simulink model "Tires"  (R2023a)
settings: Solver=VariableStepAuto  StartTime=0.0  StopTime=10.0  RelTol=1e-3
undefined symbols (not defined in the file): C, C_alpha_f, C_r, E, e_p0, F_zf, l_f, l_r, n_st
settings Model: Creator=Tan_Tram  LastModifiedBy=Tan_Tram

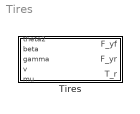
== system Tires ==
  Tires : Subsystem

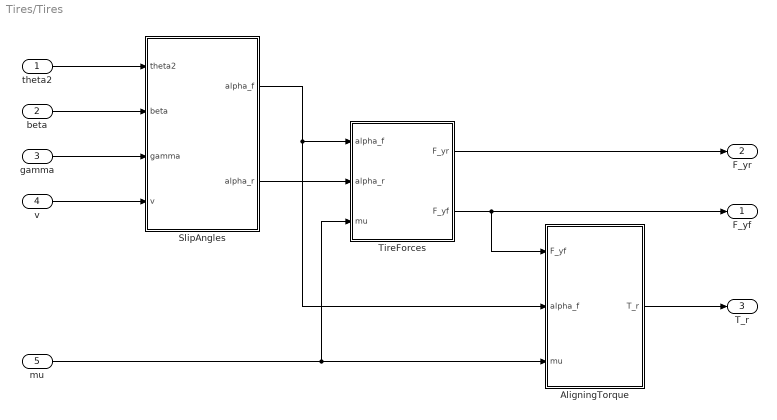
== system Tires/Tires ==
  theta2 : Inport
  beta : Inport  Port=2
  gamma : Inport  Port=3
  v : Inport  Port=4
  mu : Inport  Port=5
  AligningTorque : Subsystem
  SlipAngles : Subsystem
  TireForces : Subsystem
  F_yf : Outport
  F_yr : Outport  Port=2
  T_r : Outport  Port=3
  wires:
  v/1 -> SlipAngles/4(v)
  gamma/1 -> SlipAngles/3(gamma)
  TireForces/2(F_yf) -> F_yf/1, AligningTorque/1(F_yf)
  beta/1 -> SlipAngles/2(beta)
  theta2/1 -> SlipAngles/1(theta2)
  SlipAngles/2(alpha_r) -> TireForces/2(alpha_r)
  SlipAngles/1(alpha_f) -> TireForces/1(alpha_f), AligningTorque/2(alpha_f)
  mu/1 -> AligningTorque/3(mu), TireForces/3(mu)
  TireForces/1(F_yr) -> F_yr/1
  AligningTorque/1(T_r) -> T_r/1

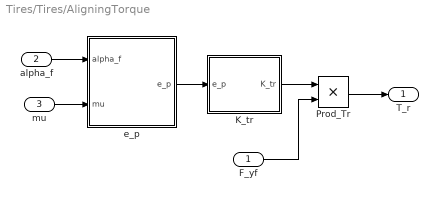
== system Tires/Tires/AligningTorque ==
  F_yf : Inport
  alpha_f : Inport  Port=2
  mu : Inport  Port=3
  K_tr : Subsystem
  Prod_Tr : Product  Inputs=**
  e_p : Subsystem
  T_r : Outport
  wires:
  F_yf/1 -> Prod_Tr/2
  Prod_Tr/1 -> T_r/1
  alpha_f/1 -> e_p/1(alpha_f)
  mu/1 -> e_p/2(mu)
  e_p/1(e_p) -> K_tr/1(e_p)
  K_tr/1(K_tr) -> Prod_Tr/1

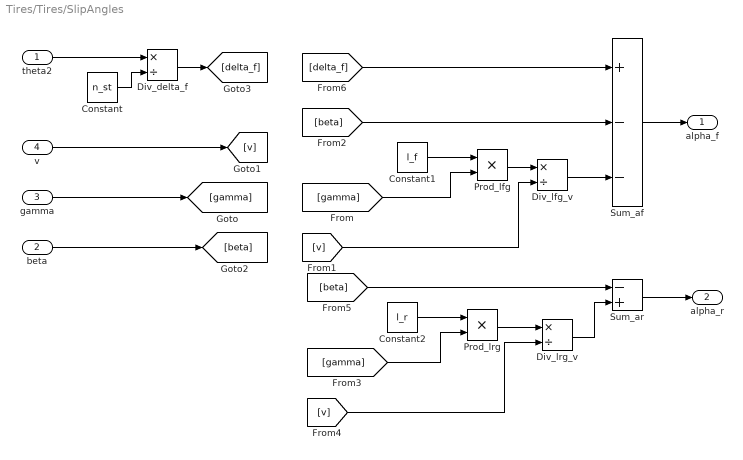
== system Tires/Tires/SlipAngles ==
  theta2 : Inport
  beta : Inport  Port=2
  gamma : Inport  Port=3
  v : Inport  Port=4
  Constant : Constant  Value=n_st
  Constant1 : Constant  Value=l_f
  Constant2 : Constant  Value=l_r
  Div_delta_f : Product  Inputs=*/
  Div_lfg_v : Product  Inputs=*/
  Div_lrg_v : Product  Inputs=*/
  Prod_lfg : Product  Inputs=**
  Prod_lrg : Product  Inputs=**
  Sum_af : Sum  Inputs=+--
  Sum_ar : Sum  Inputs=-+
  alpha_f : Outport
  alpha_r : Outport  Port=2
  wires:
  beta/1 -> [beta]
  Div_lrg_v/1 -> Sum_ar/2
  Constant2/1 -> Prod_lrg/1
  Div_lfg_v/1 -> Sum_af/3
  Constant1/1 -> Prod_lfg/1
  gamma/1 -> [gamma]
  [gamma] -> Prod_lfg/2
  v/1 -> [v]
  [gamma] -> Prod_lrg/2
  Sum_ar/1 -> alpha_r/1
  [v] -> Div_lrg_v/2
  Prod_lfg/1 -> Div_lfg_v/1
  [v] -> Div_lfg_v/2
  Prod_lrg/1 -> Div_lrg_v/1
  Sum_af/1 -> alpha_f/1
  [beta] -> Sum_af/2
  [beta] -> Sum_ar/1
  [delta_f] -> Sum_af/1
  Div_delta_f/1 -> [delta_f]
  Constant/1 -> Div_delta_f/2
  theta2/1 -> Div_delta_f/1

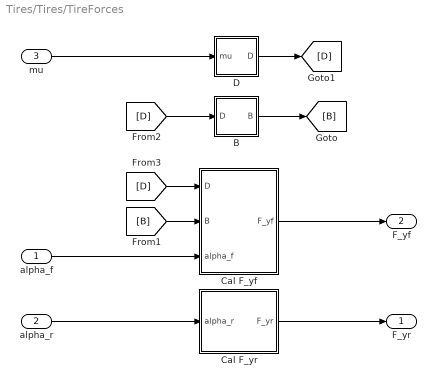
== system Tires/Tires/TireForces ==
  alpha_f : Inport
  alpha_r : Inport  Port=2
  mu : Inport  Port=3
  B : Subsystem
  Cal F_yf : Subsystem
  Cal F_yr : Subsystem
  D : Subsystem
  F_yr : Outport
  F_yf : Outport  Port=2
  wires:
  mu/1 -> D/1(mu)
  D/1(D) -> [D]
  [D] -> B/1(D)
  alpha_r/1 -> Cal F_yr/1(alpha_r)
  Cal F_yr/1(F_yr) -> F_yr/1
  B/1(B) -> [B]
  alpha_f/1 -> Cal F_yf/3(alpha_f)
  Cal F_yf/1(F_yf) -> F_yf/1
  [B] -> Cal F_yf/2(B)
  [D] -> Cal F_yf/1(D)

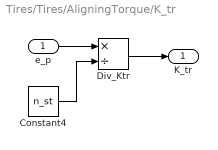
== system Tires/Tires/AligningTorque/K_tr ==
  e_p : Inport
  Constant4 : Constant  Value=n_st
  Div_Ktr : Product  Inputs=*/
  K_tr : Outport
  wires:
  Div_Ktr/1 -> K_tr/1
  e_p/1 -> Div_Ktr/1
  Constant4/1 -> Div_Ktr/2

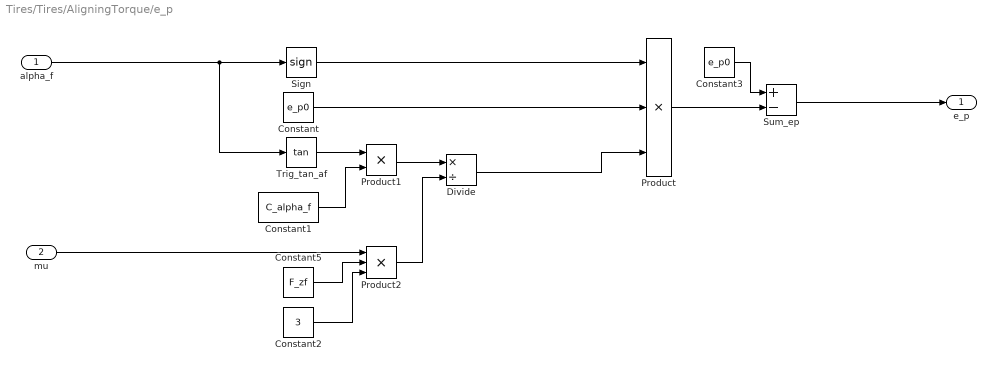
== system Tires/Tires/AligningTorque/e_p ==
  alpha_f : Inport
  mu : Inport  Port=2
  Constant : Constant  Value=e_p0
  Constant1 : Constant  Value=C_alpha_f
  Constant2 : Constant  Value=3
  Constant3 : Constant  Value=e_p0
  Constant5 : Constant  Value=F_zf
  Divide : Product  Inputs=*/
  Product : Product  Inputs=3
  Product1 : Product
  Product2 : Product  Inputs=***
  Sign : Signum
  Sum_ep : Sum  Inputs=+-
  Trig_tan_af : Trigonometry  Operator=tan
  e_p : Outport
  wires:
  Constant/1 -> Product/2
  Product1/1 -> Divide/1
  alpha_f/1 -> Sign/1, Trig_tan_af/1
  Constant1/1 -> Product1/2
  mu/1 -> Product2/1
  Trig_tan_af/1 -> Product1/1
  Constant5/1 -> Product2/2
  Constant3/1 -> Sum_ep/1
  Product/1 -> Sum_ep/2
  Constant2/1 -> Product2/3
  Divide/1 -> Product/3
  Product2/1 -> Divide/2
  Sign/1 -> Product/1
  Sum_ep/1 -> e_p/1

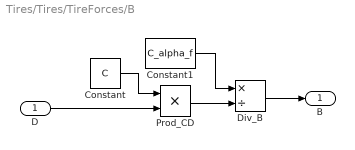
== system Tires/Tires/TireForces/B ==
  D : Inport
  Constant : Constant  Value=C
  Constant1 : Constant  Value=C_alpha_f
  Div_B : Product  Inputs=*/
  Prod_CD : Product  Inputs=**
  B : Outport
  wires:
  Div_B/1 -> B/1
  Prod_CD/1 -> Div_B/2
  Constant1/1 -> Div_B/1
  Constant/1 -> Prod_CD/1
  D/1 -> Prod_CD/2

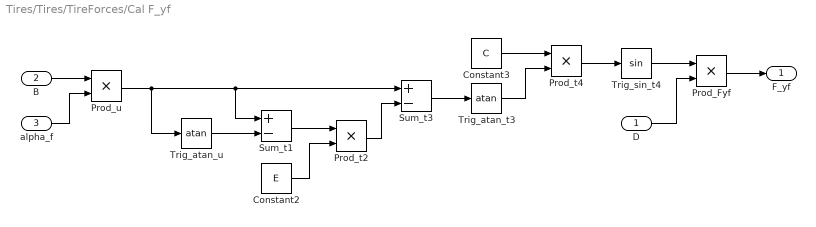
== system Tires/Tires/TireForces/Cal F_yf ==
  D : Inport
  B : Inport  Port=2
  alpha_f : Inport  Port=3
  Constant2 : Constant  Value=E
  Constant3 : Constant  Value=C
  Prod_Fyf : Product  Inputs=**
  Prod_t2 : Product  Inputs=**
  Prod_t4 : Product  Inputs=**
  Prod_u : Product  Inputs=**
  Sum_t1 : Sum  Inputs=+-
  Sum_t3 : Sum  Inputs=+-
  Trig_atan_t3 : Trigonometry  Operator=atan
  Trig_atan_u : Trigonometry  Operator=atan
  Trig_sin_t4 : Trigonometry
  F_yf : Outport
  wires:
  alpha_f/1 -> Prod_u/2
  B/1 -> Prod_u/1
  Sum_t3/1 -> Trig_atan_t3/1
  Trig_sin_t4/1 -> Prod_Fyf/1
  Sum_t1/1 -> Prod_t2/1
  Prod_t2/1 -> Sum_t3/2
  Trig_atan_t3/1 -> Prod_t4/2
  Prod_u/1 -> Sum_t1/1, Sum_t3/1, Trig_atan_u/1
  Prod_Fyf/1 -> F_yf/1
  Constant2/1 -> Prod_t2/2
  Trig_atan_u/1 -> Sum_t1/2
  Constant3/1 -> Prod_t4/1
  Prod_t4/1 -> Trig_sin_t4/1
  D/1 -> Prod_Fyf/2

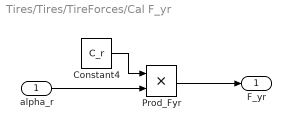
== system Tires/Tires/TireForces/Cal F_yr ==
  alpha_r : Inport
  Constant4 : Constant  Value=C_r
  Prod_Fyr : Product  Inputs=**
  F_yr : Outport
  wires:
  Constant4/1 -> Prod_Fyr/1
  Prod_Fyr/1 -> F_yr/1
  alpha_r/1 -> Prod_Fyr/2

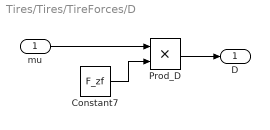
== system Tires/Tires/TireForces/D ==
  mu : Inport
  Constant7 : Constant  Value=F_zf
  Prod_D : Product  Inputs=**
  D : Outport
  wires:
  mu/1 -> Prod_D/1
  Prod_D/1 -> D/1
  Constant7/1 -> Prod_D/2
